simulink model "autosar_swc_pedal_sensor"  (R2022b)
settings: Solver=FixedStepDiscrete  StartTime=0.0  StopTime=10.0  FixedStep=0.005  RelTol=1e-3
model workspace (MATLAB code in the model file):
  | SetpointPercent_LkupTbl = Simulink.LookupTable;
  | SetpointPercent_LkupTbl.Table.DataType = 'single';
  | SetpointPercent_LkupTbl.Table.FieldName = 'Table';
  | SetpointPercent_LkupTbl.Table.Value = ...
  |   [0 10 20 30 40 50 60 70 80 90 100];
  | SetpointPercent_LkupTbl.BreakpointsSpecification = 'Explicit values';
  | SetpointPercent_LkupTbl.SupportTunableSize = false;
  | SetpointPercent_LkupTbl.Breakpoints.DataType = 'single';
  | SetpointPercent_LkupTbl.Breakpoints.FieldName = 'BP1';
  | SetpointPercent_LkupTbl.Breakpoints.Value = ...
  |   single(linspace(170, 985, 11));
  | SetpointPercent_LkupTbl.Breakpoints.TunableSizeName = 'N1';
  | SetpointPercent_LkupTbl.StructTypeInfo.Name = 'MyStruct';
  | SetpointPercent_LkupTbl.StructTypeInfo.HeaderFileName = 'Rte_Type.h';
undefined symbols (not defined in the file): TPSPercentBkpt, TPSPercentTbl
settings Model: Creator=The MathWorks, Inc.  LastModifiedBy=The MathWorks, Inc.
settings SolverCC: AlgebraicLoopSolver=TrustRegion  MaxZcPerStep=1
settings DataIOCC: SaveFormat=StructureWithTime  ReturnWorkspaceOutputs=off
settings OptimizationCC: DefaultParameterBehavior=Inlined  PassReuseOutputArgsAs=Individual arguments  ZeroExternalMemoryAtStartup=off  ZeroInternalMemoryAtStartup=off  EfficientTunableParamExpr=on
settings DebuggingCC: ParameterTunabilityLossMsg=error  UnconnectedInputMsg=warning  UnconnectedOutputMsg=warning  UnconnectedLineMsg=warning  SFMachineParentedDataDiag=warning  ArithmeticOperatorsInVariantConditions=warning
settings ModelReferenceCC: EnableRefExpFcnMdlSchedulingChecks=on
settings SFSimCC: SimUseLocalCustomCode=off  MATLABDynamicMemAlloc=off  CustomCodeUndefinedFunction=UseInterfaceOnly
settings RTWCC: Description=AUTOSAR  SystemTargetFile=autosar.tlc  GenCodeOnly=on  TemplateMakefile=ert_default_tmf  GenerateReport=on  RTWUseLocalCustomCode=off  IncludeHyperlinkInReport=on  LaunchReport=on  GenerateTraceInfo=on  GenerateTraceReport=on  GenerateTraceReportSl=on  GenerateTraceReportSf=on  GenerateTraceReportEml=on
settings CodeAppCC: ForceParamTrailComments=on  IgnoreCustomStorageClasses=off  OperatorAnnotations=on  SimulinkDataObjDesc=on  SFDataObjDesc=on  InsertBlockDesc=on
settings STFCustomTargetCC: TargetLangStandard=C99 (ISO)  MultiwordLength=256  ParMdlRefBuildCompliant=on  CompOptLevelCompliant=on  IncludeMdlTerminateFcn=off  CombineOutputUpdateFcns=on  SuppressErrorStatus=on  ERTCustomFileBanners=on  SupportNonFinite=off  SupportComplex=off  SupportContinuousTime=off  SupportNonInlinedSFcns=off  RemoveResetFunc=on  MATLABClassNameForMDSCustomization=Simulink.SoftwareTarget.ERTCustomization  CPPClassGenCompliant=on  AutosarCompliant=on  UseToolchainInfoCompliant=on  LookupTableObjectStructAxisOrder=2,1,3,4,...  LUTObjectStructOrderEvenSpacing=Size,Table,Breakpoints  SystemTargetFile=autosar.tlc
settings ERTTargetCC: TargetLangStandard=C99 (ISO)  ConcurrentExecutionCompliant=off  IncludeMdlTerminateFcn=off  SuppressErrorStatus=on  SupportNonFinite=off  SupportComplex=off  ModelStepFunctionPrototypeControlCompliant=off  AutosarCompliant=on  LookupTableObjectStructAxisOrder=2,1,3,4,...  LUTObjectStructOrderEvenSpacing=Size,Table,Breakpoints  InlinedParameterPlacement=NonHierarchical  ERTCustomFileTemplate=example_file_process.tlc

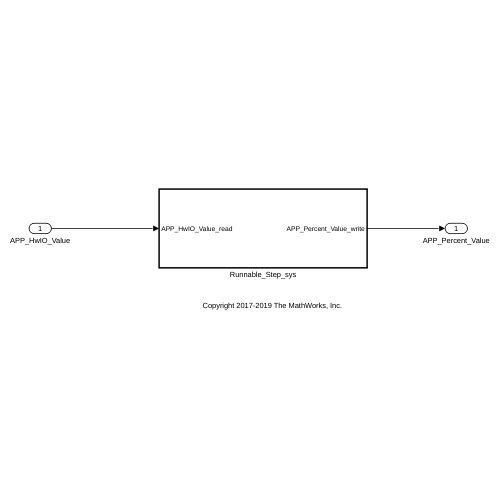
[thumbnail: Simulink's stored preview of the top-level diagram]
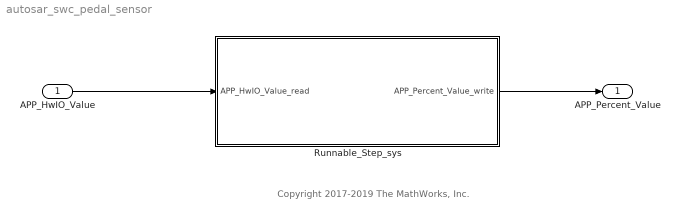
== system autosar_swc_pedal_sensor ==
  note: Copyright 2017-2019 The MathWorks, Inc.
  APP_HwIO_Value : Inport  OutDataTypeStr=uint16  PortDimensions=1
  Runnable_Step_sys : Subsystem  TreatAsAtomicUnit=on  SystemSampleTime=0.005
  APP_Percent_Value : Outport  OutDataTypeStr=single  PortDimensions=1  VectorParamsAs1DForOutWhenUnconnected=off
  wires:
  APP_HwIO_Value/1 -> Runnable_Step_sys/1(APP_HwIO_Value_read)
  Runnable_Step_sys/1(APP_Percent_Value_write) -> APP_Percent_Value/1

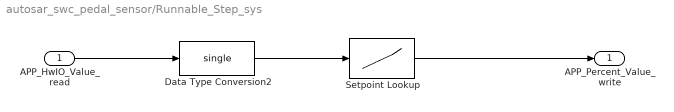
== system autosar_swc_pedal_sensor/Runnable_Step_sys ==
  APP_HwIO_Value_read : Inport
  Data Type Conversion2 : DataTypeConversion  OutDataTypeStr=single  SaturateOnIntegerOverflow=off  RndMeth=Floor
  Setpoint Lookup : Lookup_n-D  NumberOfTableDimensions=1  DataSpecification=Lookup table object  LookupTableObject=SetpointPercent_LkupTbl  BreakpointsForDimension1=TPSPercentBkpt  BreakpointsForDimension1DataTypeStr=single  IndexSearchMethod=Linear search  Table=TPSPercentTbl  TableDataTypeStr=single  ExtrapMethod=Clip  InternalRulePriority=Speed  OutDataTypeStr=single  RndMeth=Simplest
  APP_Percent_Value_write : Outport  VectorParamsAs1DForOutWhenUnconnected=off
  wires:
  APP_HwIO_Value_read/1 -> Data Type Conversion2/1
  Setpoint Lookup/1 -> APP_Percent_Value_write/1
  Data Type Conversion2/1 -> Setpoint Lookup/1
